simulink model "Brakes"  (R2020a)
settings: Solver=VariableStepAuto  StartTime=0.0  StopTime=10.0  RelTol=1e-3
settings Model: Creator=Matthew  LastModifiedBy=Matthew

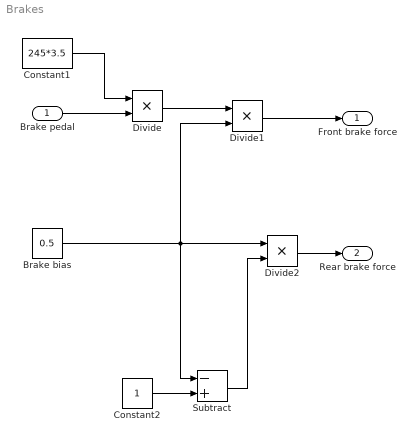
== system Brakes ==
  Brake pedal : Inport
  Brake bias : Constant  Value=0.5
  Constant1 : Constant  Value=245*3.5
  Constant2 : Constant
  Divide : Product  Inputs=**
  Divide1 : Product  Inputs=**
  Divide2 : Product  Inputs=**
  Subtract : Sum  Inputs=-+
  Front brake force : Outport
  Rear brake force : Outport  Port=2
  wires:
  Brake pedal/1 -> Divide/2
  Constant1/1 -> Divide/1
  Divide/1 -> Divide1/1
  Brake bias/1 -> Subtract/1, Divide1/2, Divide2/1
  Divide1/1 -> Front brake force/1
  Constant2/1 -> Subtract/2
  Divide2/1 -> Rear brake force/1
  Subtract/1 -> Divide2/2
